simulink model "V2_ROS2Simulink"  (R2023b)
settings: Solver=FixedStepAuto  StartTime=0.0  StopTime=inf  RelTol=1e-3
libraries: robotlib x14
settings Model: Creator=Renzhaofu  LastModifiedBy=Renzhaofu
settings OptimizationCC: EnhancedBackFolding=on  PassReuseOutputArgsAs=Individual arguments  ZeroExternalMemoryAtStartup=off  ZeroInternalMemoryAtStartup=off  MaxStackSize=64  OptimizeBlockOrder=speed  DifferentSizesBufferReuse=on  OptimizationCustomize=off  EfficientTunableParamExpr=on
settings DebuggingCC: ParameterTunabilityLossMsg=error
settings HardwareCC: ProdBitPerPointer=32  ProdBitPerSizeT=32  ProdBitPerPtrDiffT=32  ProdLargestAtomicFloat=None  ProdIntDivRoundTo=Undefined  ProdEndianess=Unspecified  ProdWordSize=32  ProdHWDeviceType=Generic->Unspecified (assume 32-bit Generic)
settings SFSimCC: MATLABDynamicMemAlloc=off
settings RTWCC: Description=Embedded Coder  SystemTargetFile=ert.tlc  HardwareBoard=Robot Operating System (ROS)  TLCOptions="-aInlineSetEventsForThisBaseRateFcn=TLC_FALSE -aSuppressMultiTaskScheduler=TLC_FALSE  -aRateBasedStepFcn=0"  TemplateMakefile=ert_default_tmf  Toolchain=Catkin  TargetLang=C++
settings CodeAppCC: ForceParamTrailComments=on  IgnoreCustomStorageClasses=off  OperatorAnnotations=on  SimulinkDataObjDesc=on  SFDataObjDesc=on  InsertBlockDesc=on

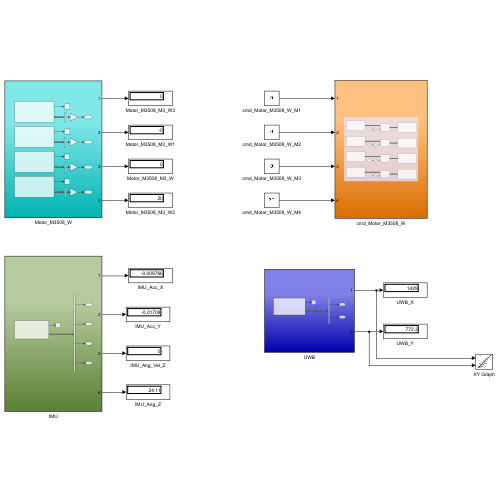
[thumbnail: Simulink's stored preview of the top-level diagram]
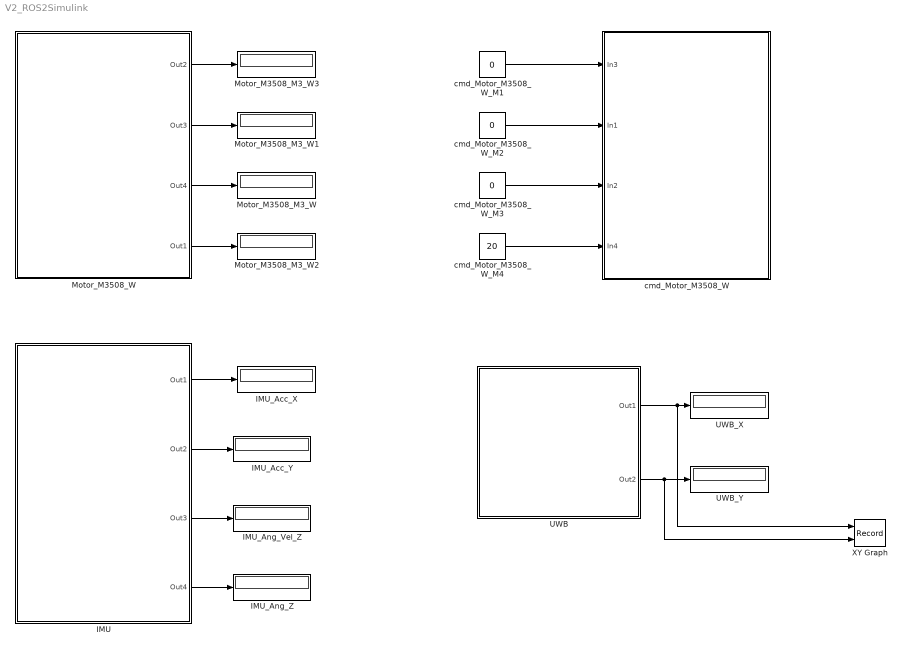
== system V2_ROS2Simulink ==
  IMU : Subsystem
  IMU_Acc_X : Display
  IMU_Acc_Y : Display
  IMU_Ang_Vel_Z : Display
  IMU_Ang_Z : Display
  Motor_M3508_M3_W{,1..3} (4 alike) : Display
  Motor_M3508_W : Subsystem
  UWB : Subsystem
  "UWB_X " : Display
  UWB_Y : Display
  XY Graph : Record  FileSettingsInternal="{\"entries\":[{\"content\":{\"excelSettings\":{\"content\":{},\"type\":\"Streamout.ExcelSettings\"}},\"type\":\"Streamout.FileSettingStorage\",\"uuid\":\"\"}],\"packageUris\":[\"http:\\/\\/schema.mathworks.com\\/mf0\\/streamout_blocks\\/R2020a\"],\"version\":\"1.0\"}"  Layout=[1 1]  SignalsInternal="{\"entries\":[{\"content\":{\"signals\":[{\"content\":{\"blockPath\":[],\"dimensions\":[1],\"domain\":\"\",\"lineColor\":\"#4dbeee\",\"port\":1,\"sid\":[\"\"],\"signalID\":42616,\"signalName\":\"UWB:1\"},\"type\":\"RecordBlkView.Signal\",\"uuid\":\"\"},{\"content\":{\"blockPath\":[],\"dimensions\":[1],\"domain\":\"\",\"lineColor\":\"#a2142f\",\"port\":2,\"sid\":[\"\"],\"signalID\":42620,\"signalName\":\"UWB:2\"},\"type\":\"RecordBlkView.Signal\",\"uuid\":\"\"}]},\"type\":\"RecordBlkView.InputSignals\",\"uuid\":\"\"}],\"packageUris\":[\"http:\\/\\/schema.mathworks.com\\/mf0\\/streamout_blocks\\/R2020a\"],\"version\":\"1.0\"}"  VisualizationBindings="{\"xyplotplugin\":{\"info\":[{\"series\":[],\"subplotID\":1}]}}"  CompatibilityTag=XY
  cmd_Motor_M3508_W : Subsystem
  cmd_Motor_M3508_W_M1 : Constant  Value=0  OutDataTypeStr=single
  cmd_Motor_M3508_W_M2 : Constant  Value=0  OutDataTypeStr=single
  cmd_Motor_M3508_W_M3 : Constant  Value=0  OutDataTypeStr=single
  cmd_Motor_M3508_W_M4 : Constant  Value=20  OutDataTypeStr=single
  wires:
  cmd_Motor_M3508_W_M1/1 -> cmd_Motor_M3508_W/1(In3)
  cmd_Motor_M3508_W_M2/1 -> cmd_Motor_M3508_W/2(In1)
  cmd_Motor_M3508_W_M3/1 -> cmd_Motor_M3508_W/3(In2)
  cmd_Motor_M3508_W_M4/1 -> cmd_Motor_M3508_W/4(In4)
  Motor_M3508_W/3(Out4) -> Motor_M3508_M3_W/1
  Motor_M3508_W/2(Out3) -> Motor_M3508_M3_W1/1
  Motor_M3508_W/1(Out2) -> Motor_M3508_M3_W3/1
  Motor_M3508_W/4(Out1) -> Motor_M3508_M3_W2/1
  IMU/1(Out1) -> IMU_Acc_X/1
  IMU/2(Out2) -> IMU_Acc_Y/1
  IMU/3(Out3) -> IMU_Ang_Vel_Z/1
  IMU/4(Out4) -> IMU_Ang_Z/1
  UWB/1(Out1) -> XY Graph/1, "UWB_X "/1
  UWB/2(Out2) -> XY Graph/2, UWB_Y/1

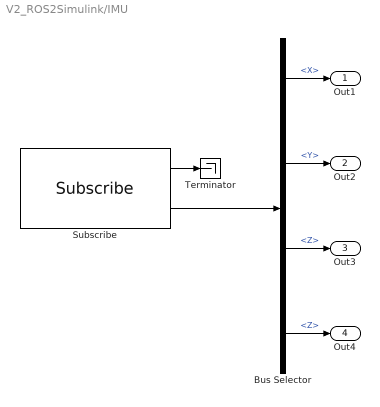
== system V2_ROS2Simulink/IMU ==
  Bus Selector : BusSelector  OutputSignals=LinearAcceleration.X,LinearAcceleration.Y,AngularVelocity.Z,Orientation.Z
  Subscribe : robotlib/Subscribe  topicSource=Select from ROS network  topic=/IMU_Topic  messageType=sensor_msgs/Imu  SampleTime=0.1  legacyBusStruct=off  messageQueueLength=1
  Terminator : Terminator
  Out1 : Outport
  Out2 : Outport  Port=2
  Out3 : Outport  Port=3
  Out4 : Outport  Port=4
  wires:
  Bus Selector/3 -> Out3/1  "<Z>"
  Subscribe/2 -> Bus Selector/1
  Subscribe/1 -> Terminator/1
  Bus Selector/4 -> Out4/1  "<Z>"
  Bus Selector/2 -> Out2/1  "<Y>"
  Bus Selector/1 -> Out1/1  "<X>"

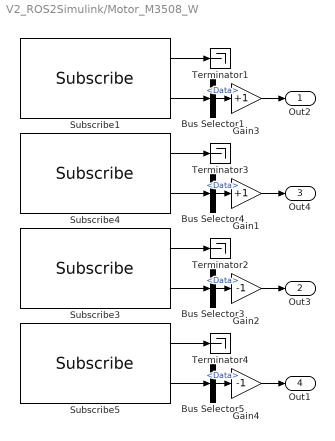
== system V2_ROS2Simulink/Motor_M3508_W ==
  Bus Selector{1,3..5} (4 alike) : BusSelector  OutputSignals=Data
  Gain1 : Gain  Gain=+1
  Gain2 : Gain  Gain=-1
  Gain3 : Gain  Gain=+1
  Gain4 : Gain  Gain=-1
  Subscribe1 : robotlib/Subscribe  topicSource=Select from ROS network  topic=/Motor_M3508_M1_W_Topic  messageType=std_msgs/Float32  SampleTime=0.1  legacyBusStruct=off  messageQueueLength=1
  Subscribe3 : robotlib/Subscribe  topicSource=Select from ROS network  topic=/Motor_M3508_M2_W_Topic  messageType=std_msgs/Float32  SampleTime=0.1  legacyBusStruct=off  messageQueueLength=1
  Subscribe4 : robotlib/Subscribe  topicSource=Select from ROS network  topic=/Motor_M3508_M3_W_Topic  messageType=std_msgs/Float32  SampleTime=0.1  legacyBusStruct=off  messageQueueLength=1
  Subscribe5 : robotlib/Subscribe  topicSource=Select from ROS network  topic=/Motor_M3508_M4_W_Topic  messageType=std_msgs/Float32  SampleTime=0.1  legacyBusStruct=off  messageQueueLength=1
  Terminator{1..4} (4 alike) : Terminator
  Out2 : Outport
  Out3 : Outport  Port=2
  Out4 : Outport  Port=3
  Out1 : Outport  Port=4
  wires:
  Subscribe5/2 -> Bus Selector5/1
  Subscribe1/1 -> Terminator1/1
  Subscribe1/2 -> Bus Selector1/1
  Subscribe3/1 -> Terminator2/1
  Subscribe4/1 -> Terminator3/1
  Subscribe4/2 -> Bus Selector4/1
  Subscribe3/2 -> Bus Selector3/1
  Subscribe5/1 -> Terminator4/1
  Gain3/1 -> Out2/1
  Bus Selector1/1 -> Gain3/1  "<Data>"
  Bus Selector5/1 -> Gain4/1  "<Data>"
  Bus Selector3/1 -> Gain2/1  "<Data>"
  Bus Selector4/1 -> Gain1/1  "<Data>"
  Gain1/1 -> Out4/1
  Gain2/1 -> Out3/1
  Gain4/1 -> Out1/1

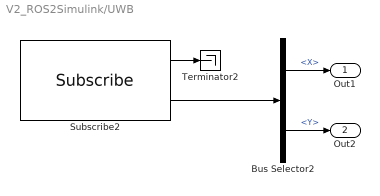
== system V2_ROS2Simulink/UWB ==
  Bus Selector2 : BusSelector  OutputSignals=X,Y
  Subscribe2 : robotlib/Subscribe  topicSource=Select from ROS network  topic=/UWB_Topic  messageType=geometry_msgs/Point  SampleTime=0.001  legacyBusStruct=off  messageQueueLength=1
  Terminator2 : Terminator
  Out1 : Outport
  Out2 : Outport  Port=2
  wires:
  Bus Selector2/1 -> Out1/1  "<X>"
  Subscribe2/2 -> Bus Selector2/1
  Subscribe2/1 -> Terminator2/1
  Bus Selector2/2 -> Out2/1  "<Y>"

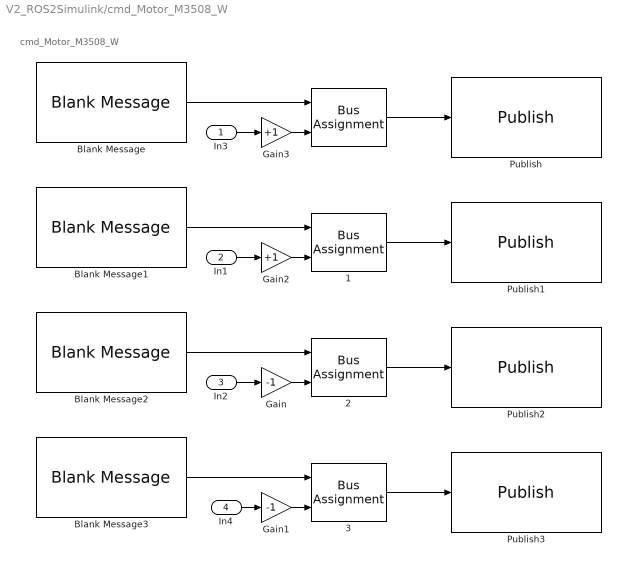
== system V2_ROS2Simulink/cmd_Motor_M3508_W ==
  note: cmd_Motor_M3508_W
  In3 : Inport
  In1 : Inport  Port=2
  In2 : Inport  Port=3
  In4 : Inport  Port=4
   {,1..3} (4 alike) : BusAssignment  AssignedSignals=Data
  Blank Message{,1..3} (4 alike) : robotlib/Blank Message  messageClass=Message  entityType=std_msgs/Float32  messageType=std_msgs/Float32  SampleTime=inf  legacyBusStruct=off
  Gain : Gain  Gain=-1
  Gain1 : Gain  Gain=-1
  Gain2 : Gain  Gain=+1
  Gain3 : Gain  Gain=+1
  Publish : robotlib/Publish  topicSource=Select from ROS network  topic=/cmd_Motor_M3508_M1_W  messageType=std_msgs/Float32  legacyBusStruct=off  messageQueueLength=1
  Publish1 : robotlib/Publish  topicSource=Select from ROS network  topic=/cmd_Motor_M3508_M2_W  messageType=std_msgs/Float32  legacyBusStruct=off  messageQueueLength=1
  Publish2 : robotlib/Publish  topicSource=Select from ROS network  topic=/cmd_Motor_M3508_M3_W  messageType=std_msgs/Float32  legacyBusStruct=off  messageQueueLength=1
  Publish3 : robotlib/Publish  topicSource=Select from ROS network  topic=/cmd_Motor_M3508_M4_W  messageType=std_msgs/Float32  legacyBusStruct=off  messageQueueLength=1
  wires:
  Blank Message/1 -> " "/1
  " 3"/1 -> Publish3/1
  " 2"/1 -> Publish2/1
  In3/1 -> Gain3/1
  Gain2/1 -> " 1"/2
  Blank Message3/1 -> " 3"/1
  " "/1 -> Publish/1
  Blank Message2/1 -> " 2"/1
  In2/1 -> Gain/1
  Gain/1 -> " 2"/2
  Gain3/1 -> " "/2
  " 1"/1 -> Publish1/1
  Blank Message1/1 -> " 1"/1
  In1/1 -> Gain2/1
  Gain1/1 -> " 3"/2
  In4/1 -> Gain1/1
